simulink model "FullState_HOSMO_UKF_STC_Half_Car_02_noised"  (R2022a)
settings: Solver=ode4  StartTime=0.0  StopTime=5  FixedStep=1e-4  RelTol=1e-3
undefined symbols (not defined in the file): DiscIntNeverNeededParam
libraries: simulink x5, sharedTrackingLibrary x1
settings Model: Creator=user  LastModifiedBy=user

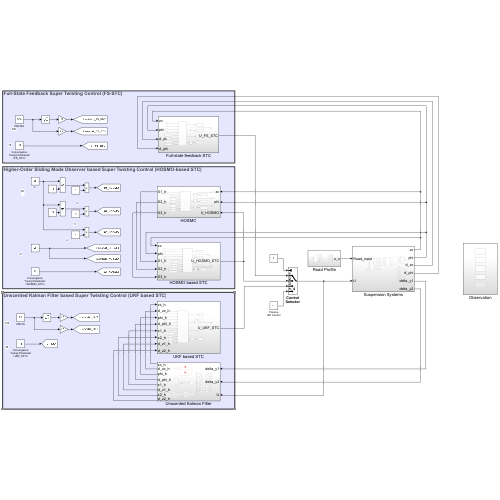
[thumbnail: Simulink's stored preview of the top-level diagram]
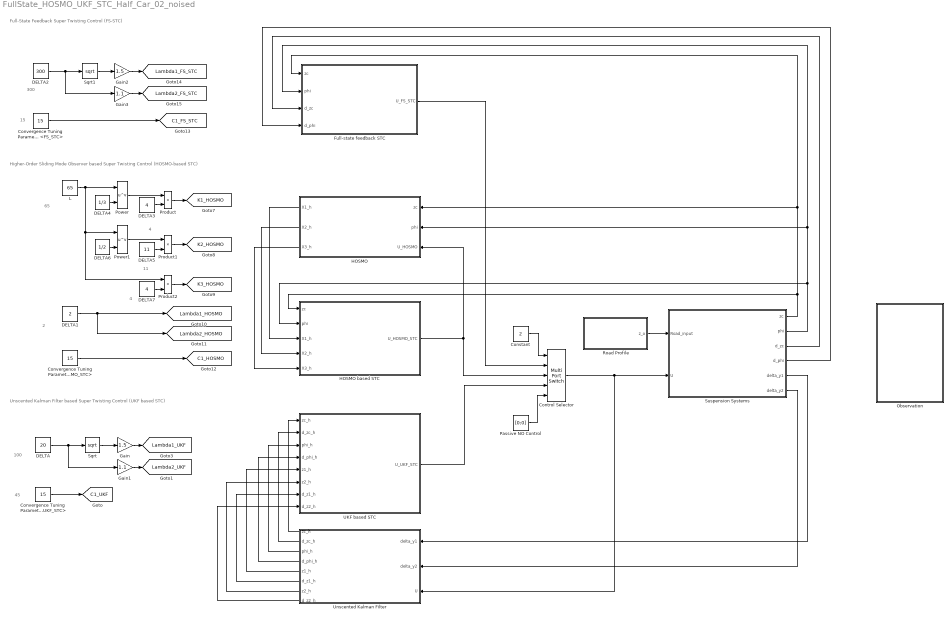
== system FullState_HOSMO_UKF_STC_Half_Car_02_noised ==
  note: 4
  note: 11
  note: 4
  note: 45
  note: 100
  note: 15
  note: 300
  note: 2
  note: 65
  note: Unscented Kalman Filter based Super Twisting Control (UKF based STC)
  note: Higher-Order Sliding Mode Observer based Super Twisting Control (HOSMO-based STC)
  note: Full-State Feedback Super Twisting Control (FS-STC)
  Constant : Constant  Value=2
  Control Selector : MultiPortSwitch  Inputs=4  SaturateOnIntegerOverflow=off  InputSameDT=off
  Convergence Tuning Parameter <FS_STC> : Constant  Value=15
  Convergence Tuning Parameter <HOSMO_STC> : Constant  Value=15
  Convergence Tuning Parameter <UKF_STC> : Constant  Value=15
  DELTA : Constant  Value=20
  DELTA1 : Constant  Value=2
  DELTA2 : Constant  Value=300
  DELTA3 : Constant  Value=4
  DELTA4 : Constant  Value=1/3
  DELTA5 : Constant  Value=11
  DELTA6 : Constant  Value=1/2
  DELTA7 : Constant  Value=4
  Full-state feedback STC : Subsystem
  Gain : Gain  Gain=1.5
  Gain1 : Gain  Gain=1.1
  Gain2 : Gain  Gain=1.5
  Gain3 : Gain  Gain=1.1
  HOSMO : Subsystem
  HOSMO based STC : Subsystem
  L : Constant  Value=65
  Observation : Subsystem
  Passive NO Control : Constant  Value=[0;0]
  Power : Math  Operator=pow
  Power1 : Math  Operator=pow
  Product : Product
  Product1 : Product
  Product2 : Product
  Road Profile : Subsystem
  Sqrt : Sqrt
  Sqrt1 : Sqrt
  Suspension Systems : Subsystem
  UKF based STC : Subsystem
  Unscented Kalman Filter : Subsystem
  tag scope: C1_FS_STC=global, C1_HOSMO=global, C1_UKF=global, K1_HOSMO=global, K2_HOSMO=global, K3_HOSMO=global, Lambda1_FS_STC=global, Lambda1_HOSMO=global, Lambda1_UKF=global, Lambda2_FS_STC=global, Lambda2_HOSMO=global, Lambda2_UKF=global
  wires:
  Road Profile/1(z_o) -> Suspension Systems/1(Road_input)
  Suspension Systems/5(delta_y1) -> Unscented Kalman Filter/1(delta_y1)
  Suspension Systems/6(delta_y2) -> Unscented Kalman Filter/2(delta_y2)
  Control Selector/1 -> Unscented Kalman Filter/3(U), Suspension Systems/2(U)
  Unscented Kalman Filter/1(zc_h) -> UKF based STC/1(zc_h)
  Unscented Kalman Filter/2(d_zc_h) -> UKF based STC/2(d_zc_h)
  Unscented Kalman Filter/3(phi_h) -> UKF based STC/3(phi_h)
  Unscented Kalman Filter/4(d_phi_h) -> UKF based STC/4(d_phi_h)
  Unscented Kalman Filter/6(d_z1_h) -> UKF based STC/7(d_z1_h)
  Unscented Kalman Filter/8(d_z2_h) -> UKF based STC/8(d_z2_h)
  Unscented Kalman Filter/7(z2_h) -> UKF based STC/6(z2_h)
  Unscented Kalman Filter/5(z1_h) -> UKF based STC/5(z1_h)
  Constant/1 -> Control Selector/1
  Passive NO Control/1 -> Control Selector/5
  UKF based STC/1(U_UKF_STC) -> Control Selector/4
  HOSMO based STC/1(U_HOSMO_STC) -> Control Selector/3, HOSMO/3(U_HOSMO)
  HOSMO/1(X1_h) -> HOSMO based STC/3(X1_h)
  HOSMO/2(X2_h) -> HOSMO based STC/4(X2_h)
  HOSMO/3(X3_h) -> HOSMO based STC/5(X3_h)
  Suspension Systems/1(zc) -> Full-state feedback STC/1(zc), HOSMO/1(zc), HOSMO based STC/1(zc)
  Suspension Systems/2(phi) -> Full-state feedback STC/2(phi), HOSMO/2(phi), HOSMO based STC/2(phi)
  DELTA/1 -> Sqrt/1, Gain1/1
  Convergence Tuning Parameter <UKF_STC>/1 -> [C1_UKF]
  Gain/1 -> [Lambda1_UKF]
  Gain1/1 -> [Lambda2_UKF]
  Sqrt/1 -> Gain/1
  Convergence Tuning Parameter <HOSMO_STC>/1 -> [C1_HOSMO]
  DELTA1/1 -> [Lambda2_HOSMO], [Lambda1_HOSMO]
  L/1 -> Product2/1, Power1/1, Power/1
  Product/1 -> [K1_HOSMO]
  DELTA4/1 -> Power/2
  Power/1 -> Product/1
  DELTA3/1 -> Product/2
  DELTA5/1 -> Product1/2
  Power1/1 -> Product1/1
  DELTA6/1 -> Power1/2
  Product1/1 -> [K2_HOSMO]
  DELTA7/1 -> Product2/2
  Product2/1 -> [K3_HOSMO]
  Convergence Tuning Parameter <FS_STC>/1 -> [C1_FS_STC]
  Sqrt1/1 -> Gain2/1
  DELTA2/1 -> Sqrt1/1, Gain3/1
  Gain2/1 -> [Lambda1_FS_STC]
  Gain3/1 -> [Lambda2_FS_STC]
  Full-state feedback STC/1(U_FS_STC) -> Control Selector/2
  Suspension Systems/3(d_zc) -> Full-state feedback STC/3(d_zc)
  Suspension Systems/4(d_phi) -> Full-state feedback STC/4(d_phi)

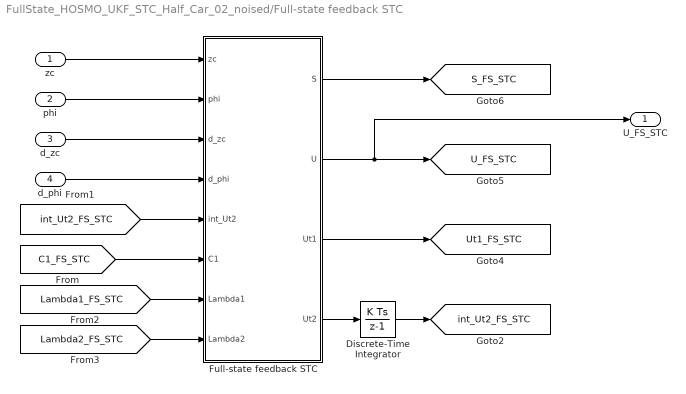
== system FullState_HOSMO_UKF_STC_Half_Car_02_noised/Full-state feedback STC ==
  zc : Inport
  phi : Inport  Port=2
  d_zc : Inport  Port=3
  d_phi : Inport  Port=4
  Discrete-Time Integrator : DiscreteIntegrator  InitialCondition=[0;0]  SampleTime=-1  ICPrevOutput=DiscIntNeverNeededParam  ICPrevScaledInput=DiscIntNeverNeededParam
  Full-state feedback STC : MATLAB Function  TreatAsAtomicUnit=on
  U_FS_STC : Outport
  tag scope: S_FS_STC=global, U_FS_STC=global, Ut1_FS_STC=global, int_Ut2_FS_STC=global
  wires:
  d_phi/1 -> Full-state feedback STC/4(d_phi)
  d_zc/1 -> Full-state feedback STC/3(d_zc)
  Full-state feedback STC/3(Ut1) -> [Ut1_FS_STC]
  [Lambda2_FS_STC] -> Full-state feedback STC/8(Lambda2)
  zc/1 -> Full-state feedback STC/1(zc)
  Discrete-Time Integrator/1 -> [int_Ut2_FS_STC]
  Full-state feedback STC/4(Ut2) -> Discrete-Time Integrator/1
  Full-state feedback STC/2(U) -> U_FS_STC/1, [U_FS_STC]
  phi/1 -> Full-state feedback STC/2(phi)
  Full-state feedback STC/1(S) -> [S_FS_STC]
  [Lambda1_FS_STC] -> Full-state feedback STC/7(Lambda1)
  [int_Ut2_FS_STC] -> Full-state feedback STC/5(int_Ut2)
  [C1_FS_STC] -> Full-state feedback STC/6(C1)

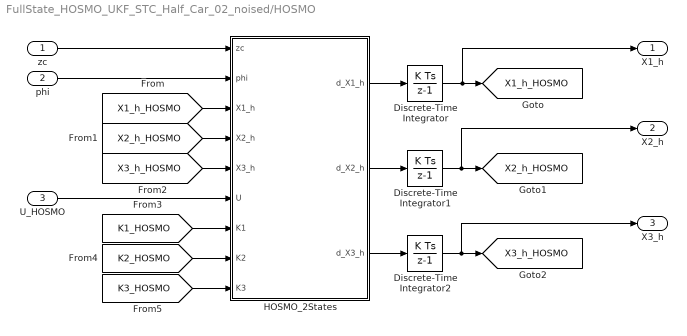
== system FullState_HOSMO_UKF_STC_Half_Car_02_noised/HOSMO ==
  zc : Inport
  phi : Inport  Port=2
  U_HOSMO : Inport  Port=3
  Discrete-Time Integrator : DiscreteIntegrator  InitialCondition=[0;0]  SampleTime=-1  ICPrevOutput=DiscIntNeverNeededParam  ICPrevScaledInput=DiscIntNeverNeededParam
  Discrete-Time Integrator1 : DiscreteIntegrator  InitialCondition=[0;0]  SampleTime=-1  ICPrevOutput=DiscIntNeverNeededParam  ICPrevScaledInput=DiscIntNeverNeededParam
  Discrete-Time Integrator2 : DiscreteIntegrator  InitialCondition=[0;0]  SampleTime=-1  ICPrevOutput=DiscIntNeverNeededParam  ICPrevScaledInput=DiscIntNeverNeededParam
  HOSMO_2States : MATLAB Function  TreatAsAtomicUnit=on
  X1_h : Outport
  X2_h : Outport  Port=2
  X3_h : Outport  Port=3
  tag scope: X1_h_HOSMO=global, X2_h_HOSMO=global, X3_h_HOSMO=global
  wires:
  HOSMO_2States/2(d_X2_h) -> Discrete-Time Integrator1/1
  [K1_HOSMO] -> HOSMO_2States/7(K1)
  Discrete-Time Integrator1/1 -> X2_h/1, [X2_h_HOSMO]
  [K2_HOSMO] -> HOSMO_2States/8(K2)
  [K3_HOSMO] -> HOSMO_2States/9(K3)
  [X1_h_HOSMO] -> HOSMO_2States/3(X1_h)
  [X3_h_HOSMO] -> HOSMO_2States/5(X3_h)
  Discrete-Time Integrator/1 -> X1_h/1, [X1_h_HOSMO]
  HOSMO_2States/1(d_X1_h) -> Discrete-Time Integrator/1
  HOSMO_2States/3(d_X3_h) -> Discrete-Time Integrator2/1
  zc/1 -> HOSMO_2States/1(zc)
  [X2_h_HOSMO] -> HOSMO_2States/4(X2_h)
  Discrete-Time Integrator2/1 -> X3_h/1, [X3_h_HOSMO]
  phi/1 -> HOSMO_2States/2(phi)
  U_HOSMO/1 -> HOSMO_2States/6(U)

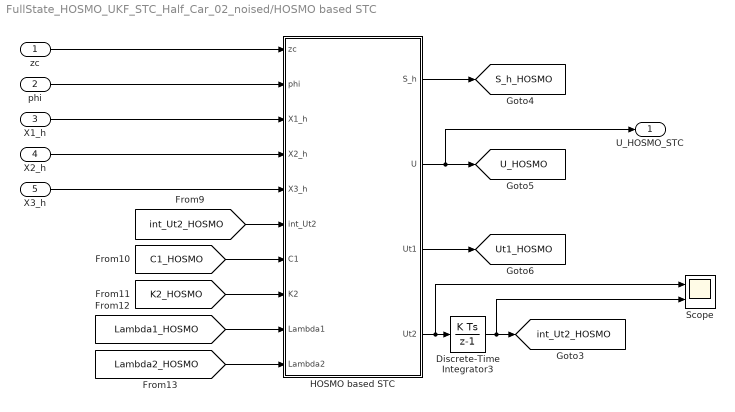
== system FullState_HOSMO_UKF_STC_Half_Car_02_noised/HOSMO based STC ==
  zc : Inport
  phi : Inport  Port=2
  X1_h : Inport  Port=3
  X2_h : Inport  Port=4
  X3_h : Inport  Port=5
  Discrete-Time Integrator3 : DiscreteIntegrator  InitialCondition=[0;0]  SampleTime=-1  ICPrevOutput=DiscIntNeverNeededParam  ICPrevScaledInput=DiscIntNeverNeededParam
  HOSMO based STC : MATLAB Function  TreatAsAtomicUnit=on
  Scope : Scope  NumInputPorts=2
  U_HOSMO_STC : Outport
  tag scope: S_h_HOSMO=global, U_HOSMO=global, Ut1_HOSMO=global, int_Ut2_HOSMO=global
  wires:
  Discrete-Time Integrator3/1 -> Scope/2, [int_Ut2_HOSMO]
  [Lambda1_HOSMO] -> HOSMO based STC/9(Lambda1)
  HOSMO based STC/1(S_h) -> [S_h_HOSMO]
  HOSMO based STC/2(U) -> U_HOSMO_STC/1, [U_HOSMO]
  HOSMO based STC/3(Ut1) -> [Ut1_HOSMO]
  X3_h/1 -> HOSMO based STC/5(X3_h)
  [Lambda2_HOSMO] -> HOSMO based STC/10(Lambda2)
  X1_h/1 -> HOSMO based STC/3(X1_h)
  phi/1 -> HOSMO based STC/2(phi)
  X2_h/1 -> HOSMO based STC/4(X2_h)
  [int_Ut2_HOSMO] -> HOSMO based STC/6(int_Ut2)
  [K2_HOSMO] -> HOSMO based STC/8(K2)
  [C1_HOSMO] -> HOSMO based STC/7(C1)
  HOSMO based STC/4(Ut2) -> Scope/1, Discrete-Time Integrator3/1
  zc/1 -> HOSMO based STC/1(zc)

== system FullState_HOSMO_UKF_STC_Half_Car_02_noised/Observation ==
  FullState_STC : Subsystem
  HOSMO_STC : Subsystem
  OVERALL : Subsystem
  To Workspace : Subsystem  Commented=on
  UKF_STC : Subsystem

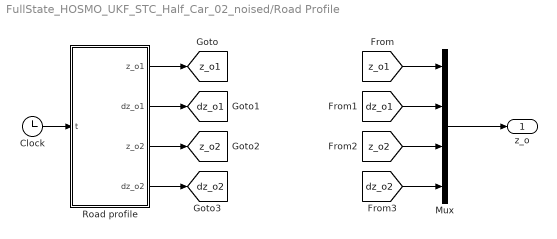
== system FullState_HOSMO_UKF_STC_Half_Car_02_noised/Road Profile ==
  Clock : Clock
  Mux : Mux
  Road profile : MATLAB Function  TreatAsAtomicUnit=on
  z_o : Outport
  tag scope: dz_o1=global, dz_o2=global, z_o1=global, z_o2=global
  wires:
  Road profile/3(z_o2) -> [z_o2]
  Mux/1 -> z_o/1
  Road profile/1(z_o1) -> [z_o1]
  Clock/1 -> Road profile/1(t)
  Road profile/4(dz_o2) -> [dz_o2]
  Road profile/2(dz_o1) -> [dz_o1]
  [z_o1] -> Mux/1
  [dz_o1] -> Mux/2
  [dz_o2] -> Mux/4
  [z_o2] -> Mux/3

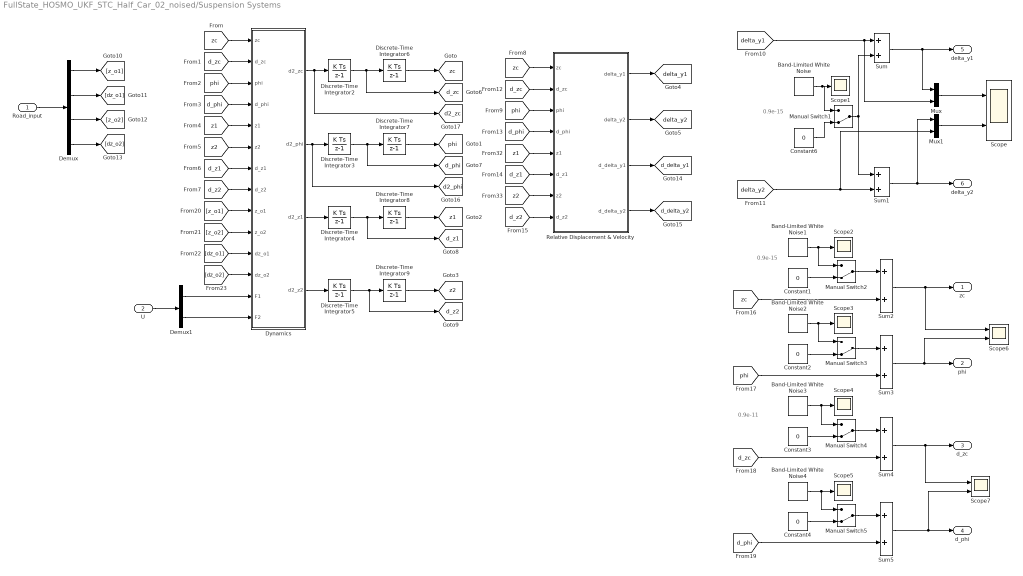
== system FullState_HOSMO_UKF_STC_Half_Car_02_noised/Suspension Systems ==
  note: 0.9e-11
  note: 0.9e-15
  note: 0.9e-15
  Road_input : Inport
  U : Inport  Port=2
  Band-Limited White Noise : simulink/Sources/Band-Limited White Noise  Cov=0.9e-15  Ts=1e-4  seed=[23341]
  Band-Limited White Noise1 : simulink/Sources/Band-Limited White Noise  Cov=0.9e-15  Ts=1e-4  seed=[23341]
  Band-Limited White Noise2 : simulink/Sources/Band-Limited White Noise  Cov=0.9e-15  Ts=1e-4  seed=[23341]
  Band-Limited White Noise3 : simulink/Sources/Band-Limited White Noise  Cov=0.9e-11  Ts=1e-4  seed=[23341]
  Band-Limited White Noise4 : simulink/Sources/Band-Limited White Noise  Cov=0.9e-11  Ts=1e-4  seed=[23341]
  Constant{1..4,6} (5 alike) : Constant  Value=0
  Demux : Demux
  Demux1 : Demux  Outputs=2
  Discrete-Time Integrator{2..9} (8 alike) : DiscreteIntegrator  SampleTime=-1  ICPrevOutput=DiscIntNeverNeededParam  ICPrevScaledInput=DiscIntNeverNeededParam
  Dynamics : MATLAB Function  TreatAsAtomicUnit=on
  Manual Switch{1..5} (5 alike) : ManualSwitch  CurrentSetting=0
  Mux : Mux  Inputs=2
  Mux1 : Mux  Inputs=2
  Relative Displacement & Velocity : MATLAB Function  TreatAsAtomicUnit=on
  Scope : Scope  NumInputPorts=2
  Scope{1..5} (5 alike) : Scope
  Scope6 : Scope  NumInputPorts=2
  Scope7 : Scope  NumInputPorts=2
  Sum{,1..5} (6 alike) : Sum
  zc : Outport
  phi : Outport  Port=2
  d_zc : Outport  Port=3
  d_phi : Outport  Port=4
  delta_y1 : Outport  Port=5
  delta_y2 : Outport  Port=6
  tag scope: d2_phi=global, d2_zc=global, d_delta_y1=global, d_delta_y2=global, d_phi=global, d_z1=global, d_z2=global, d_zc=global, delta_y1=global, delta_y2=global, phi=global, z1=global, z2=global, zc=global
  wires:
  Dynamics/4(d2_z2) -> Discrete-Time Integrator5/1
  Discrete-Time Integrator2/1 -> [d_zc], Discrete-Time Integrator6/1
  Relative Displacement & Velocity/1(delta_y1) -> [delta_y1]
  Discrete-Time Integrator4/1 -> [d_z1], Discrete-Time Integrator8/1
  [z1] -> Dynamics/5(z1)
  [dz_o2] -> Dynamics/12(dz_o2)
  Discrete-Time Integrator3/1 -> [d_phi], Discrete-Time Integrator7/1
  [zc] -> Relative Displacement & Velocity/1(zc)
  Dynamics/2(d2_phi) -> [d2_phi], Discrete-Time Integrator3/1
  [d_phi] -> Dynamics/4(d_phi)
  Discrete-Time Integrator5/1 -> [d_z2], Discrete-Time Integrator9/1
  Discrete-Time Integrator7/1 -> [phi]
  [z_o2] -> Dynamics/10(z_o2)
  [z1] -> Relative Displacement & Velocity/5(z1)
  Discrete-Time Integrator6/1 -> [zc]
  Dynamics/3(d2_z1) -> Discrete-Time Integrator4/1
  Discrete-Time Integrator8/1 -> [z1]
  [d_zc] -> Dynamics/2(d_zc)
  [phi] -> Dynamics/3(phi)
  Road_input/1 -> Demux/1
  [z2] -> Dynamics/6(z2)
  [zc] -> Dynamics/1(zc)
  [z_o1] -> Dynamics/9(z_o1)
  Dynamics/1(d2_zc) -> [d2_zc], Discrete-Time Integrator2/1
  [d_z1] -> Dynamics/7(d_z1)
  [dz_o1] -> Dynamics/11(dz_o1)
  Relative Displacement & Velocity/2(delta_y2) -> [delta_y2]
  [d_z2] -> Dynamics/8(d_z2)
  Discrete-Time Integrator9/1 -> [z2]
  [phi] -> Relative Displacement & Velocity/3(phi)
  [z2] -> Relative Displacement & Velocity/7(z2)
  Demux/1 -> [z_o1]
  Demux/2 -> [dz_o1]
  Demux/3 -> [z_o2]
  Demux/4 -> [dz_o2]
  [d_zc] -> Relative Displacement & Velocity/2(d_zc)
  [d_phi] -> Relative Displacement & Velocity/4(d_phi)
  [d_z1] -> Relative Displacement & Velocity/6(d_z1)
  [d_z2] -> Relative Displacement & Velocity/8(d_z2)
  Relative Displacement & Velocity/3(d_delta_y1) -> [d_delta_y1]
  Relative Displacement & Velocity/4(d_delta_y2) -> [d_delta_y2]
  Demux1/1 -> Dynamics/13(F1)
  Demux1/2 -> Dynamics/14(F2)
  U/1 -> Demux1/1
  Manual Switch1/1 -> Sum1/1, Sum/2
  Constant6/1 -> Manual Switch1/2
  Sum1/1 -> Mux1/1, delta_y2/1
  Sum/1 -> Mux/1, delta_y1/1
  [delta_y1] -> Sum/1, Mux/2
  Band-Limited White Noise/1 -> Manual Switch1/1, Scope1/1
  [delta_y2] -> Mux1/2, Sum1/2
  Mux/1 -> Scope/1
  Mux1/1 -> Scope/2
  [zc] -> Sum2/2
  Band-Limited White Noise1/1 -> Manual Switch2/1, Scope2/1
  Constant1/1 -> Manual Switch2/2
  Manual Switch2/1 -> Sum2/1
  Sum2/1 -> Scope6/1, zc/1
  Sum3/1 -> Scope6/2, phi/1
  Manual Switch3/1 -> Sum3/1
  Constant2/1 -> Manual Switch3/2
  Band-Limited White Noise2/1 -> Scope3/1, Manual Switch3/1
  [phi] -> Sum3/2
  Band-Limited White Noise3/1 -> Scope4/1, Manual Switch4/1
  Constant3/1 -> Manual Switch4/2
  Manual Switch4/1 -> Sum4/1
  [d_zc] -> Sum4/2
  Sum4/1 -> Scope7/1, d_zc/1
  Manual Switch5/1 -> Sum5/1
  Constant4/1 -> Manual Switch5/2
  Band-Limited White Noise4/1 -> Manual Switch5/1, Scope5/1
  [d_phi] -> Sum5/2
  Sum5/1 -> Scope7/2, d_phi/1

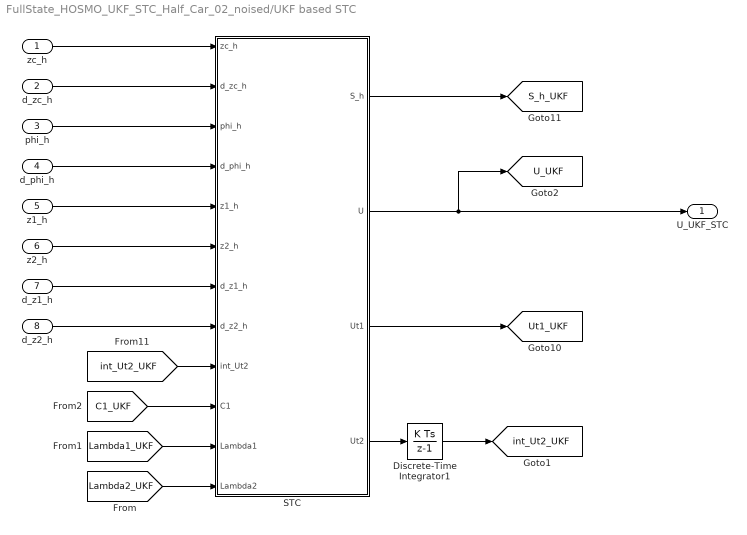
== system FullState_HOSMO_UKF_STC_Half_Car_02_noised/UKF based STC ==
  zc_h : Inport
  d_zc_h : Inport  Port=2
  phi_h : Inport  Port=3
  d_phi_h : Inport  Port=4
  z1_h : Inport  Port=5
  z2_h : Inport  Port=6
  d_z1_h : Inport  Port=7
  d_z2_h : Inport  Port=8
  Discrete-Time Integrator1 : DiscreteIntegrator  InitialCondition=[0;0]  SampleTime=-1  ICPrevOutput=DiscIntNeverNeededParam  ICPrevScaledInput=DiscIntNeverNeededParam
  STC : MATLAB Function  TreatAsAtomicUnit=on
  U_UKF_STC : Outport
  tag scope: S_h_UKF=global, U_UKF=global, Ut1_UKF=global, int_Ut2_UKF=global
  wires:
  phi_h/1 -> STC/3(phi_h)
  STC/2(U) -> [U_UKF], U_UKF_STC/1
  d_zc_h/1 -> STC/2(d_zc_h)
  zc_h/1 -> STC/1(zc_h)
  z2_h/1 -> STC/6(z2_h)
  [Lambda2_UKF] -> STC/12(Lambda2)
  Discrete-Time Integrator1/1 -> [int_Ut2_UKF]
  STC/1(S_h) -> [S_h_UKF]
  z1_h/1 -> STC/5(z1_h)
  STC/3(Ut1) -> [Ut1_UKF]
  [Lambda1_UKF] -> STC/11(Lambda1)
  [C1_UKF] -> STC/10(C1)
  STC/4(Ut2) -> Discrete-Time Integrator1/1
  d_phi_h/1 -> STC/4(d_phi_h)
  [int_Ut2_UKF] -> STC/9(int_Ut2)
  d_z1_h/1 -> STC/7(d_z1_h)
  d_z2_h/1 -> STC/8(d_z2_h)

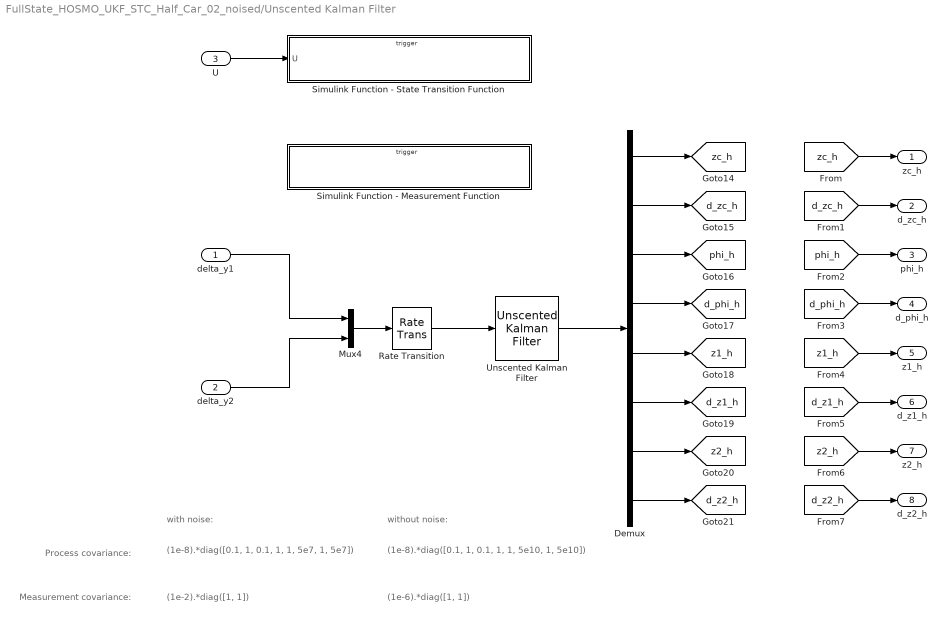
== system FullState_HOSMO_UKF_STC_Half_Car_02_noised/Unscented Kalman Filter ==
  note: Measurement covariance:
  note: (1e-6).*diag([1, 1])
  note: (1e-8).*diag([0.1, 1, 0.1, 1, 1, 5e7, 1, 5e7])
  note: (1e-2).*diag([1, 1])
  note: Process covariance:
  note: with noise:
  note: without noise:
  note: (1e-8).*diag([0.1, 1, 0.1, 1, 1, 5e10, 1, 5e10])
  delta_y1 : Inport
  delta_y2 : Inport  Port=2
  U : Inport  Port=3
  Demux : Demux  Outputs=8
  Mux4 : Mux  Inputs=2
  Rate Transition : RateTransition  InitialCondition=[0;0]  OutPortSampleTime=1e-4
  Simulink Function - Measurement Function : Subsystem  TreatAsAtomicUnit=on
  Simulink Function - State Transition Function : Subsystem  TreatAsAtomicUnit=on
  Unscented Kalman Filter : sharedTrackingLibrary/Unscented Kalman Filter  StateTransitionFcn=SuspensionStateFcn  HasAdditiveProcessNoise=Additive  ProcessNoise=(1e-8).*diag([0.1, 1, 0.1, 1, 1, 5e10, 1, 5e10])  HasTimeVaryingProcessNoise=off  HasStateTransitionFcnExtraArgument=0  InitialState=zeros(8,1)  InitialStateCovariance=diag([0, 0, 0, 0, 0, 0, 0, 0])  Alpha=1  Beta=2  Kappa=0  MeasurementFcn1=SuspensionMeasurementFcn  HasMeasurementEnablePort1=off  HasAdditiveMeasurementNoise1=Additive  MeasurementNoise1=(1e-6).*diag([1, 1])  HasTimeVaryingMeasurementNoise1=off  HasMeasurementFcnExtraArgument1=0  HasMeasurementWrapping1=off  MeasurementFcn2=myMeasurementFcn  HasMeasurementEnablePort2=off  HasAdditiveMeasurementNoise2=Additive  MeasurementNoise2=1  HasTimeVaryingMeasurementNoise2=off  HasMeasurementFcnExtraArgument2=0  HasMeasurementWrapping2=off  MeasurementFcn3=myMeasurementFcn  HasMeasurementEnablePort3=off  HasAdditiveMeasurementNoise3=Additive  MeasurementNoise3=1  HasTimeVaryingMeasurementNoise3=off  HasMeasurementFcnExtraArgument3=0  HasMeasurementWrapping3=off  MeasurementFcn4=myMeasurementFcn  HasMeasurementEnablePort4=off  HasAdditiveMeasurementNoise4=Additive  MeasurementNoise4=1  HasTimeVaryingMeasurementNoise4=off  HasMeasurementFcnExtraArgument4=0  HasMeasurementWrapping4=off  MeasurementFcn5=myMeasurementFcn  HasMeasurementEnablePort5=off  HasAdditiveMeasurementNoise5=Additive  MeasurementNoise5=1  HasTimeVaryingMeasurementNoise5=off  HasMeasurementFcnExtraArgument5=0  HasMeasurementWrapping5=off  EnableMultirate=off  StateTransitionFcnSampleTime=-1  MeasurementFcn1SampleTime=-1  MeasurementFcn2SampleTime=-1  MeasurementFcn3SampleTime=-1  MeasurementFcn4SampleTime=-1  MeasurementFcn5SampleTime=-1  UseCurrentEstimator=on  OutputStateCovariance=off  DataType=double  SampleTime=1e-4  NumberOfMeasurements=1
      settings: SourceProductBaseCode=TF,AE,PW,CT,DR,ID,LP,NV,AR,RO,RR,UV,VE
  zc_h : Outport
  d_zc_h : Outport  Port=2
  phi_h : Outport  Port=3
  d_phi_h : Outport  Port=4
  z1_h : Outport  Port=5
  d_z1_h : Outport  Port=6
  z2_h : Outport  Port=7
  d_z2_h : Outport  Port=8
  tag scope: d_phi_h=global, d_z1_h=global, d_z2_h=global, d_zc_h=global, phi_h=global, z1_h=global, z2_h=global, zc_h=global
  wires:
  Mux4/1 -> Rate Transition/1
  Demux/4 -> [d_phi_h]
  U/1 -> Simulink Function - State Transition Function/1(U)
  Demux/8 -> [d_z2_h]
  Unscented Kalman Filter/1 -> Demux/1
  Rate Transition/1 -> Unscented Kalman Filter/1
  Demux/6 -> [d_z1_h]
  Demux/5 -> [z1_h]
  Demux/2 -> [d_zc_h]
  Demux/7 -> [z2_h]
  Demux/1 -> [zc_h]
  Demux/3 -> [phi_h]
  [d_z2_h] -> d_z2_h/1
  [d_z1_h] -> d_z1_h/1
  [d_phi_h] -> d_phi_h/1
  [phi_h] -> phi_h/1
  [d_zc_h] -> d_zc_h/1
  [zc_h] -> zc_h/1
  [z1_h] -> z1_h/1
  [z2_h] -> z2_h/1
  delta_y1/1 -> Mux4/1
  delta_y2/1 -> Mux4/2

== system FullState_HOSMO_UKF_STC_Half_Car_02_noised/Observation/FullState_STC ==
  FS_STC : Scope  NumInputPorts=4
  wires:
  [Ut1_FS_STC] -> FS_STC/3  "Super twisting control 1"
  [U_FS_STC] -> FS_STC/2  "Total Control"
  [int_Ut2_FS_STC] -> FS_STC/4  "Super twisting control 2"
  [S_FS_STC] -> FS_STC/1  "Sliding Surface"

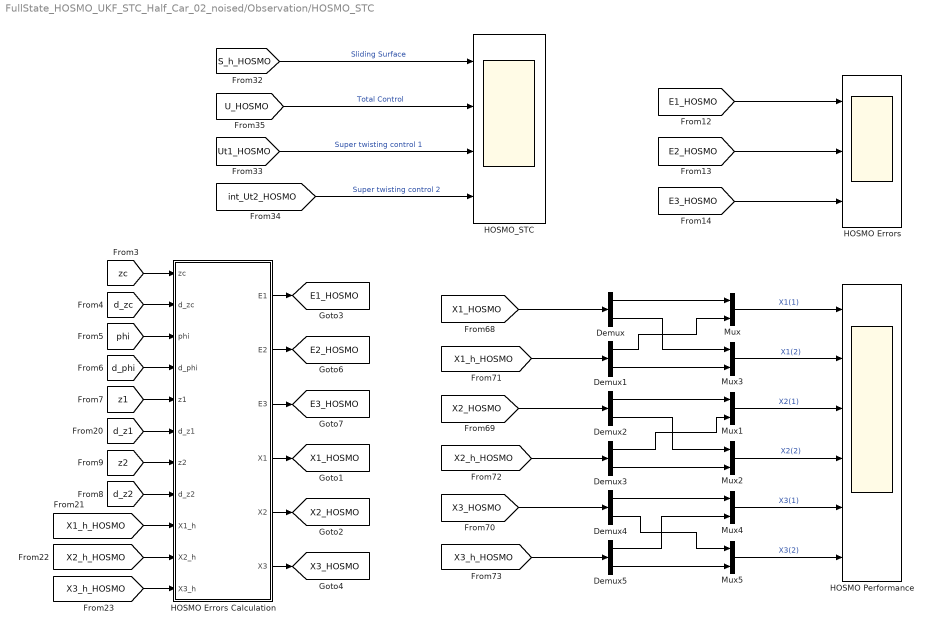
== system FullState_HOSMO_UKF_STC_Half_Car_02_noised/Observation/HOSMO_STC ==
  Demux{,1..5} (6 alike) : Demux  Outputs=2
  HOSMO Errors : Scope  NumInputPorts=3
  HOSMO Errors Calculation : MATLAB Function  TreatAsAtomicUnit=on
  HOSMO Performance : Scope  NumInputPorts=6
  HOSMO_STC : Scope  NumInputPorts=4
  Mux{,1..5} (6 alike) : Mux  Inputs=2
  tag scope: E1_HOSMO=global, E2_HOSMO=global, E3_HOSMO=global, X1_HOSMO=global, X2_HOSMO=global, X3_HOSMO=global
  wires:
  Demux1/2 -> Mux3/2
  HOSMO Errors Calculation/6(X3) -> [X3_HOSMO]
  Demux/1 -> Mux/1
  Demux5/1 -> Mux4/2
  [d_phi] -> HOSMO Errors Calculation/4(d_phi)
  [X2_HOSMO] -> Demux2/1
  HOSMO Errors Calculation/2(E2) -> [E2_HOSMO]
  Mux5/1 -> HOSMO Performance/6  "X3(2)"
  [X3_h_HOSMO] -> HOSMO Errors Calculation/11(X3_h)
  Demux/2 -> Mux3/1
  [d_z1] -> HOSMO Errors Calculation/6(d_z1)
  [d_z2] -> HOSMO Errors Calculation/8(d_z2)
  HOSMO Errors Calculation/4(X1) -> [X1_HOSMO]
  Demux2/1 -> Mux1/1
  [d_zc] -> HOSMO Errors Calculation/2(d_zc)
  HOSMO Errors Calculation/3(E3) -> [E3_HOSMO]
  [X2_h_HOSMO] -> Demux3/1
  [X1_HOSMO] -> Demux/1
  Demux2/2 -> Mux2/1
  HOSMO Errors Calculation/5(X2) -> [X2_HOSMO]
  [X3_h_HOSMO] -> Demux5/1
  Mux/1 -> HOSMO Performance/1  "X1(1)"
  Demux4/2 -> Mux5/1
  HOSMO Errors Calculation/1(E1) -> [E1_HOSMO]
  Demux4/1 -> Mux4/1
  [int_Ut2_HOSMO] -> HOSMO_STC/4  "Super twisting control 2"
  Demux5/2 -> Mux5/2
  [X1_h_HOSMO] -> Demux1/1
  [z2] -> HOSMO Errors Calculation/7(z2)
  Mux3/1 -> HOSMO Performance/2  "X1(2)"
  Mux1/1 -> HOSMO Performance/3  "X2(1)"
  Mux4/1 -> HOSMO Performance/5  "X3(1)"
  Demux3/2 -> Mux2/2
  Mux2/1 -> HOSMO Performance/4  "X2(2)"
  [U_HOSMO] -> HOSMO_STC/2  "Total Control"
  [X1_h_HOSMO] -> HOSMO Errors Calculation/9(X1_h)
  [E3_HOSMO] -> HOSMO Errors/3
  [S_h_HOSMO] -> HOSMO_STC/1  "Sliding Surface"
  [X3_HOSMO] -> Demux4/1
  [X2_h_HOSMO] -> HOSMO Errors Calculation/10(X2_h)
  Demux1/1 -> Mux/2
  [phi] -> HOSMO Errors Calculation/3(phi)
  [zc] -> HOSMO Errors Calculation/1(zc)
  [Ut1_HOSMO] -> HOSMO_STC/3  "Super twisting control 1"
  [z1] -> HOSMO Errors Calculation/5(z1)
  [E2_HOSMO] -> HOSMO Errors/2
  Demux3/1 -> Mux1/2
  [E1_HOSMO] -> HOSMO Errors/1

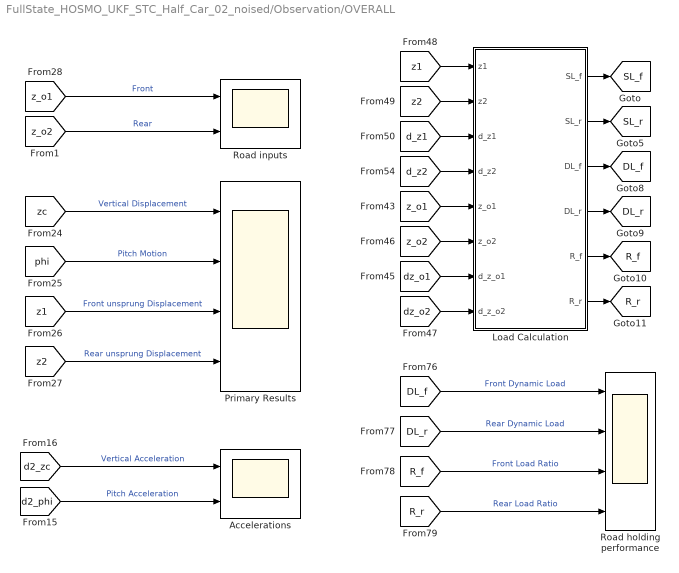
== system FullState_HOSMO_UKF_STC_Half_Car_02_noised/Observation/OVERALL ==
  Accelerations : Scope  NumInputPorts=2
  Load Calculation : MATLAB Function  TreatAsAtomicUnit=on
  Primary Results : Scope  NumInputPorts=4
  Road holding performance : Scope  NumInputPorts=4
  Road inputs : Scope  NumInputPorts=2
  tag scope: DL_f=global, DL_r=global, R_f=global, R_r=global, SL_f=global, SL_r=global
  wires:
  Load Calculation/2(SL_r) -> [SL_r]
  [DL_f] -> Road holding performance/1  "Front Dynamic Load"
  [z_o2] -> Load Calculation/6(z_o2)
  Load Calculation/6(R_r) -> [R_r]
  [z_o1] -> Load Calculation/5(z_o1)
  [d_z1] -> Load Calculation/3(d_z1)
  Load Calculation/5(R_f) -> [R_f]
  [d2_phi] -> Accelerations/2  "Pitch Acceleration"
  Load Calculation/3(DL_f) -> [DL_f]
  [zc] -> Primary Results/1  "Vertical Displacement"
  [d_z2] -> Load Calculation/4(d_z2)
  [z1] -> Load Calculation/1(z1)
  [z2] -> Load Calculation/2(z2)
  [d2_zc] -> Accelerations/1  "Vertical Acceleration"
  Load Calculation/1(SL_f) -> [SL_f]
  [z2] -> Primary Results/4  "Rear unsprung Displacement"
  [z1] -> Primary Results/3  "Front unsprung Displacement"
  [dz_o1] -> Load Calculation/7(d_z_o1)
  [R_f] -> Road holding performance/3  "Front Load Ratio"
  [phi] -> Primary Results/2  "Pitch Motion"
  [dz_o2] -> Load Calculation/8(d_z_o2)
  Load Calculation/4(DL_r) -> [DL_r]
  [z_o1] -> Road inputs/1  "Front"
  [R_r] -> Road holding performance/4  "Rear Load Ratio"
  [z_o2] -> Road inputs/2  "Rear"
  [DL_r] -> Road holding performance/2  "Rear Dynamic Load"

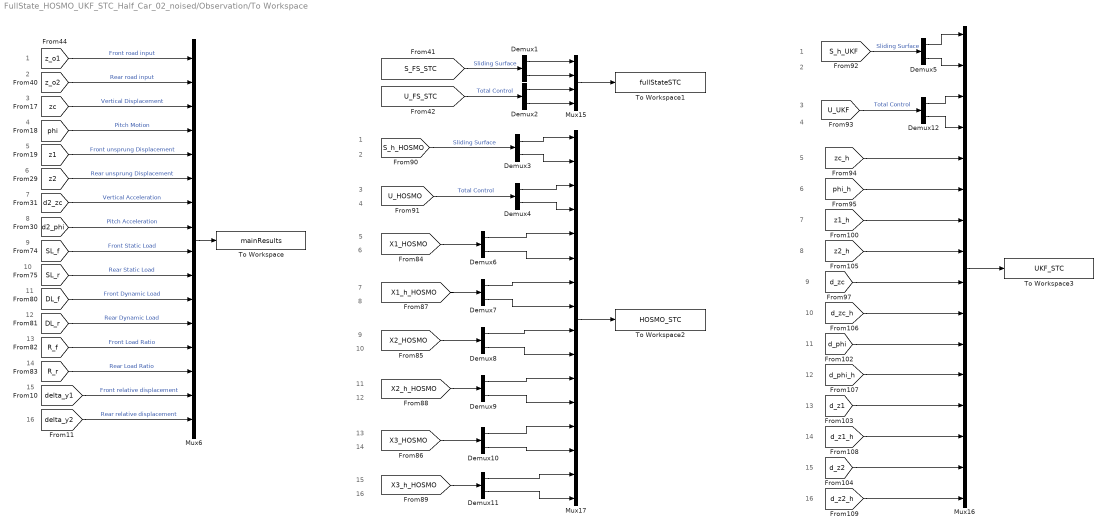
== system FullState_HOSMO_UKF_STC_Half_Car_02_noised/Observation/To Workspace ==
  note: 16
  note: 15
  note: 14
  note: 13
  note: 12
  note: 11
  note: 10
  note: 9
  note: 8
  note: 7
  note: 6
  note: 5
  note: 4
  note: 3
  note: 2
  note: 1
  note: 9
  note: 13
  note: 8
  note: 6
  note: 2
  note: 12
  note: 3
  note: 16
  note: 11
  note: 10
  note: 14
  note: 7
  note: 5
  note: 15
  note: 4
  note: 1
  note: 9
  note: 13
  note: 8
  note: 6
  note: 2
  note: 12
  note: 3
  note: 16
  note: 11
  note: 10
  note: 14
  note: 7
  note: 5
  note: 15
  note: 4
  note: 1
  Demux{1..12} (12 alike) : Demux  Outputs=2
  Mux15 : Mux
  Mux16 : Mux  Inputs=16
  Mux17 : Mux  Inputs=16
  Mux6 : Mux  Inputs=16
  To Workspace : ToWorkspace  VariableName=mainResults  SaveFormat=Structure With Time  SampleTime=-1
  To Workspace1 : ToWorkspace  VariableName=fullStateSTC  SaveFormat=Structure With Time  SampleTime=-1
  To Workspace2 : ToWorkspace  VariableName=HOSMO_STC  SaveFormat=Structure With Time  SampleTime=-1
  To Workspace3 : ToWorkspace  VariableName=UKF_STC  SaveFormat=Structure With Time  SampleTime=-1
  wires:
  [X2_h_HOSMO] -> Demux9/1
  [U_HOSMO] -> Demux4/1  "Total Control"
  [DL_r] -> Mux6/12  "Rear Dynamic Load"
  [z1_h] -> Mux16/7
  [z_o1] -> Mux6/1  "Front road input"
  [d2_phi] -> Mux6/8  "Pitch Acceleration"
  [z_o2] -> Mux6/2  "Rear road input"
  Demux10/1 -> Mux17/13
  Demux7/1 -> Mux17/7
  Mux17/1 -> To Workspace2/1
  [R_f] -> Mux6/13  "Front Load Ratio"
  Mux15/1 -> To Workspace1/1
  Demux7/2 -> Mux17/8
  [z2] -> Mux6/6  "Rear unsprung Displacement"
  [d_z1_h] -> Mux16/14
  [S_h_UKF] -> Demux5/1  "Sliding Surface"
  [d2_zc] -> Mux6/7  "Vertical Acceleration"
  Demux6/1 -> Mux17/5
  [S_h_HOSMO] -> Demux3/1  "Sliding Surface"
  [zc_h] -> Mux16/5
  Demux6/2 -> Mux17/6
  [U_FS_STC] -> Demux2/1  "Total Control"
  [d_zc_h] -> Mux16/10
  [d_z1] -> Mux16/13
  Demux9/1 -> Mux17/11
  [d_zc] -> Mux16/9
  [phi_h] -> Mux16/6
  Mux6/1 -> To Workspace/1
  [SL_f] -> Mux6/9  "Front Static Load"
  [X3_h_HOSMO] -> Demux11/1
  [phi] -> Mux6/4  "Pitch Motion"
  Demux11/2 -> Mux17/16
  [X1_h_HOSMO] -> Demux7/1
  [z1] -> Mux6/5  "Front unsprung Displacement"
  Demux11/1 -> Mux17/15
  [zc] -> Mux6/3  "Vertical Displacement"
  [S_FS_STC] -> Demux1/1  "Sliding Surface"
  [d_z2_h] -> Mux16/16
  Demux8/1 -> Mux17/9
  [SL_r] -> Mux6/10  "Rear Static Load"
  [z2_h] -> Mux16/8
  [d_z2] -> Mux16/15
  [X1_HOSMO] -> Demux6/1
  [d_phi] -> Mux16/11
  Demux8/2 -> Mux17/10
  [U_UKF] -> Demux12/1  "Total Control"
  [DL_f] -> Mux6/11  "Front Dynamic Load"
  Mux16/1 -> To Workspace3/1
  Demux10/2 -> Mux17/14
  [X2_HOSMO] -> Demux8/1
  Demux9/2 -> Mux17/12
  [R_r] -> Mux6/14  "Rear Load Ratio"
  [d_phi_h] -> Mux16/12
  [X3_HOSMO] -> Demux10/1
  [delta_y1] -> Mux6/15  "Front relative displacement"
  [delta_y2] -> Mux6/16  "Rear relative displacement"
  Demux1/1 -> Mux15/1
  Demux1/2 -> Mux15/2
  Demux2/1 -> Mux15/3
  Demux2/2 -> Mux15/4
  Demux3/1 -> Mux17/1
  Demux3/2 -> Mux17/2
  Demux4/1 -> Mux17/3
  Demux4/2 -> Mux17/4
  Demux12/2 -> Mux16/4
  Demux12/1 -> Mux16/3
  Demux5/2 -> Mux16/2
  Demux5/1 -> Mux16/1

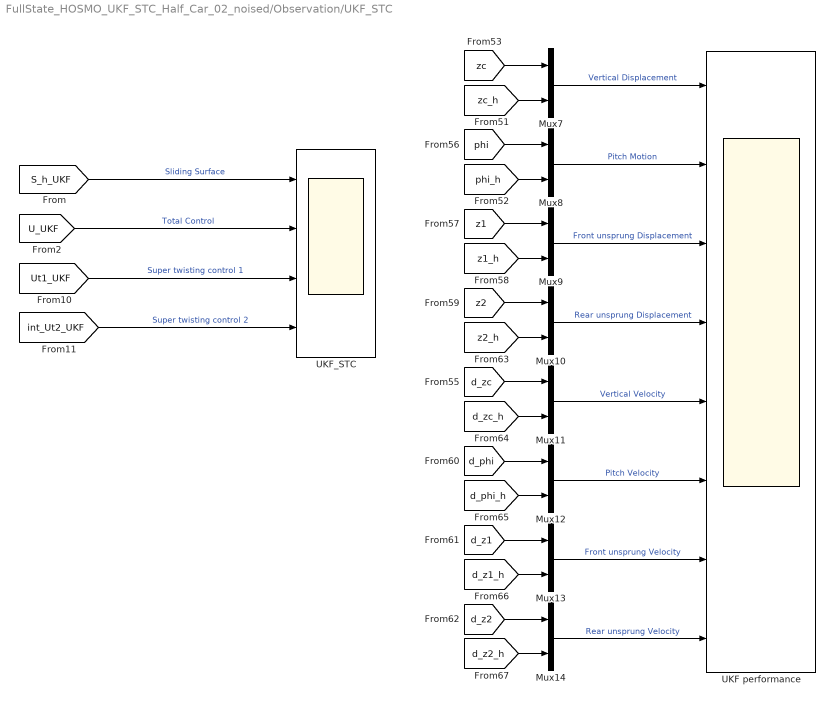
== system FullState_HOSMO_UKF_STC_Half_Car_02_noised/Observation/UKF_STC ==
  Mux{7..14} (8 alike) : Mux  Inputs=2
  UKF performance : Scope  NumInputPorts=8
  UKF_STC : Scope  NumInputPorts=4
  wires:
  Mux7/1 -> UKF performance/1  "Vertical Displacement"
  [S_h_UKF] -> UKF_STC/1  "Sliding Surface"
  [d_z1_h] -> Mux13/2
  [zc] -> Mux7/1
  Mux8/1 -> UKF performance/2  "Pitch Motion"
  [d_z1] -> Mux13/1
  [phi_h] -> Mux8/2
  [U_UKF] -> UKF_STC/2  "Total Control"
  Mux9/1 -> UKF performance/3  "Front unsprung Displacement"
  [int_Ut2_UKF] -> UKF_STC/4  "Super twisting control 2"
  [z2_h] -> Mux10/2
  [d_phi_h] -> Mux12/2
  [d_zc_h] -> Mux11/2
  Mux14/1 -> UKF performance/8  "Rear unsprung Velocity"
  [phi] -> Mux8/1
  [d_zc] -> Mux11/1
  Mux13/1 -> UKF performance/7  "Front unsprung Velocity"
  [Ut1_UKF] -> UKF_STC/3  "Super twisting control 1"
  Mux10/1 -> UKF performance/4  "Rear unsprung Displacement"
  [zc_h] -> Mux7/2
  Mux12/1 -> UKF performance/6  "Pitch Velocity"
  [d_phi] -> Mux12/1
  [z2] -> Mux10/1
  [z1_h] -> Mux9/2
  [d_z2_h] -> Mux14/2
  [d_z2] -> Mux14/1
  Mux11/1 -> UKF performance/5  "Vertical Velocity"
  [z1] -> Mux9/1

== system FullState_HOSMO_UKF_STC_Half_Car_02_noised/Unscented Kalman Filter/Simulink Function - Measurement Function ==
  SuspensionMeasurementFcn : TriggerPort  TriggerType=function-call  IsSimulinkFunction=on  FunctionName=SuspensionMeasurementFcn  VariantControl=Variant
  f(x) : MATLAB Function  TreatAsAtomicUnit=on
  x : ArgIn  DisableCoverage=on  PortDimensions=[8,1]  ArgumentName=x
  y : ArgOut  DisableCoverage=on  PortDimensions=[2,1]  ArgumentName=y
  wires:
  x/1 -> f(x)/1(X)
  f(x)/1(y) -> y/1

== system FullState_HOSMO_UKF_STC_Half_Car_02_noised/Unscented Kalman Filter/Simulink Function - State Transition Function ==
  U : Inport
  SuspensionStateFcn : TriggerPort  TriggerType=function-call  IsSimulinkFunction=on  FunctionName=SuspensionStateFcn  VariantControl=Variant
  Add : Sum
  Demux : Demux  Outputs=2
  Product : Product
  Time constant : Constant  Value=1E-4
  f(x,u) : MATLAB Function  TreatAsAtomicUnit=on
  x : ArgIn  DisableCoverage=on  PortDimensions=[8,1]  ArgumentName=x
  xNext : ArgOut  DisableCoverage=on  PortDimensions=[8,1]  ArgumentName=xNext
  wires:
  x/1 -> f(x,u)/1(X), Add/1
  Add/1 -> xNext/1
  Time constant/1 -> Product/2
  Product/1 -> Add/2
  Demux/1 -> f(x,u)/2(F1)
  Demux/2 -> f(x,u)/3(F2)
  U/1 -> Demux/1
  f(x,u)/1(Xdot) -> Product/1

== matlab function FullState_HOSMO_UKF_STC_Half_Car_02_noised/Suspension Systems/Relative Displacement & Velocity ==
  data: zc input; d_zc input; delta_y1 output; phi input; d_phi input; z1 input; d_z1 input; z2 input; delta_y2 output; d_z2 input; d_delta_y1 output; d_delta_y2 output
function [delta_y1, delta_y2, d_delta_y1, d_delta_y2] = fcn(zc, d_zc, phi, d_phi, z1, d_z1, z2, d_z2)
%% Parameters
% M = 1200; % [kg] mass of the vehicle body
% M_max = 1500; % [kg]
% M_min = 1000; % [kg]
% m_f = 100; m_r = 100; % [kg] unsprung masses of front and rear
% b_e1 = 2500; b_e2 = 2500; % [Ns/m] damping coefficient of the suspension system
% k_s1 = 15000; k_s2 = 15000; % [N/m] stiffness coefficient of the suspension system
% k_t1 = 200000; k_t2 = 200000; % [N/m] conpressibleness coefficient of the pneumatic tire
% P_s = 5*10^6; % [Pa] supply pressure
% mu = 2.32*10^8;
% C_tp = 4*10^-13; % total leakage coefficient of the piston
% V_t = 1.2*10^-3; % [m^3] total actuator volume
% V_0  = 20; % [m/s] velocity of the vehicle
% I = 600; I_max = 700; I_min = 500; % [kgm^2] mass moment of inertia
% k_nf1 = 1000; k_nr1 = 1000; % [N/m]
% b_t1 = 1000; b_t2 = 1000; % [N/m] damping coefficient of the pneumatic tire
a = 1.2; b = 1.5; % [m] distance of the suspensions to the center of mass of the vehicle body
% A = 0.006; % [m^2] ram area of the cylinder
% beta_e = 700*10^6; % [Pa] effective bulk modulus
% beta_emax = 800*10^6; % [Pa]
% beta_emin = 200*10^6; % [Pa]
%% Suspension displacements
delta_y1 = zc + a*sin(phi) - z1;
delta_y2 = zc - b*sin(phi) - z2;
d_delta_y1 = d_zc + a*d_phi*cos(phi) - d_z1;
d_delta_y2 = d_zc - b*d_phi*cos(phi) - d_z2;

== matlab function FullState_HOSMO_UKF_STC_Half_Car_02_noised/Observation/HOSMO_STC/HOSMO Errors Calculation ==
  data: zc input; d_zc input; E1 output; E2 output; E3 output; phi input; d_phi input; z1 input; d_z1 input; z2 input; d_z2 input; X1_h input; X2_h input; X3_h input; X1 output; X2 output; X3 output
function [E1, E2, E3, X1, X2, X3] = fcn(zc, d_zc, phi, d_phi, z1, d_z1, z2, d_z2, X1_h, X2_h, X3_h)
%% Parameters
M = 1200; % [kg] mass of the vehicle body
% M_max = 1500; % [kg]
% M_min = 1000; % [kg]
% m_f = 100; m_r = 100; % [kg] unsprung masses of front and rear
b_e1 = 2500; b_e2 = 2500; % [Ns/m] damping coefficient of the suspension system
k_s1 = 15000; k_s2 = 15000; % [N/m] stiffness coefficient of the suspension system
% k_t1 = 200000; k_t2 = 200000; % [N/m] conpressibleness coefficient of the pneumatic tire
% P_s = 5*10^6; % [Pa] supply pressure
% mu = 2.32*10^8;
% C_tp = 4*10^-13; % total leakage coefficient of the piston
% V_t = 1.2*10^-3; % [m^3] total actuator volume
% V_0  = 20; % [m/s] velocity of the vehicle
I = 600;
% I_max = 700; I_min = 500; % [kgm^2] mass moment of inertia
% k_nf1 = 1000; k_nr1 = 1000; % [N/m]
% b_t1 = 1000; b_t2 = 1000; % [N/m] damping coefficient of the pneumatic tire
a = 1.2; b = 1.5; % [m] distance of the suspensions to the center of mass of the vehicle body
% A = 0.006; % [m^2] ram area of the cylinder
% beta_e = 700*10^6; % [Pa] effective bulk modulus
% beta_emax = 800*10^6; % [Pa]
% beta_emin = 200*10^6; % [Pa]
%% Error Calculation
X1 = [zc; phi];
X2 = [d_zc; d_phi];
% Internal Matrices
A = [-(k_s1 + k_s2)/M, -(a*k_s1 - b*k_s2)/M; -(a*k_s1 - b*k_s2)/I, -(a^2*k_s1 + b^2*k_s2)/I];
B = [-(b_e1 + b_e2)/M, -(a*b_e1 - b*b_e2)/M; -(a*b_e1 - b*b_e2)/I, -(a^2*b_e1 + b^2*b_e2)/I];
H = A*X1 + B*X2; % actual
H_h = A*X1 + B*X2_h; % estimated
% Lumped Disturbance
d1 = (-1/M)*(-k_s1*z1 - k_s2*z2 - b_e1*d_z1 - b_e2*d_z2 + (a*k_s1 - b*k_s2)*(sin(phi)-phi) + (a*b_e1-b*b_e2)*d_phi*(cos(phi)-1));
d2 = (-1/I)*(-a*k_s1*z1 + b*k_s2*z2 - a*b_e1*d_z1 + b*b_e2*d_z2 + (a^2*k_s1 + b^2*k_s2)*(sin(phi) - phi) + (a^2*b_e1 - b^2*b_e2)*d_phi*(cos(phi)-1));
D = [d1; d2];
X3 = D + H - H_h;
% Observer estimation errors
E1 = X1 - X1_h;
E2 = X2 - X2_h;
E3 = X3 - X3_h;

== matlab function FullState_HOSMO_UKF_STC_Half_Car_02_noised/Full-state feedback STC/Full-state feedback STC ==
  data: zc input; S output; phi input; d_zc input; d_phi input; int_Ut2 input; U output; Ut1 output; Ut2 output; C1 input; Lambda1 input; Lambda2 input
function [S, U, Ut1, Ut2] = fcn(zc, phi, d_zc, d_phi, int_Ut2, C1, Lambda1, Lambda2)
%% Parameters
M = 1200; % [kg] mass of the vehicle body
% M_max = 1500; % [kg]
% M_min = 1000; % [kg]
b_e1 = 2500; b_e2 = 2500; % [Ns/m] damping coefficient of the suspension system
k_s1 = 15000; k_s2 = 15000; % [N/m] stiffness coefficient of the suspension system
I = 600; % [kgm^2] mass moment of inertia
% I_max = 700; I_min = 500;
a = 1.2; b = 1.5; % [m] distance of the suspensions to the center of mass of the vehicle body
%% Control-oriented System Dynamics
% d_X1 = X2;
% d_X2 = H + G*U + D
X1 = [zc; phi];
X2 = [d_zc; d_phi];
% Internal Matrices
A = [-(k_s1 + k_s2)/M, -(a*k_s1 - b*k_s2)/M; -(a*k_s1 - b*k_s2)/I, -(a^2*k_s1 + b^2*k_s2)/I];
B = [-(b_e1 + b_e2)/M, -(a*b_e1 - b*b_e2)/M; -(a*b_e1 - b*b_e2)/I, -(a^2*b_e1 + b^2*b_e2)/I];
H = A*X1 + B*X2; % actual
% Control Matrix
G = [1/M, 1/M; a/I, -b/I];
% Sliding surface
S = C1*X1 + X2;
% Control law
Ut1 = Lambda1.*nthroot(abs(S),2).*sign(S);
Ut2 = Lambda2.*sign(S);
U = G\(-C1.*X2 - H - Ut1 - int_Ut2);

== matlab function FullState_HOSMO_UKF_STC_Half_Car_02_noised/Unscented Kalman Filter/Simulink Function - Measurement Function/f(x) ==
  data: X input; y output
function y = fy(X)
%% Parameters
% M = 1200; % [kg] mass of the vehicle body
% M_max = 1500; % [kg]
% M_min = 1000; % [kg]
% m_f = 100; m_r = 100; % [kg] unsprung masses of front and rear
% b_e1 = 2500; b_e2 = 2500; % [Ns/m] damping coefficient of the suspension system
% k_s1 = 15000; k_s2 = 15000; % [N/m] stiffness coefficient of the suspension system
% k_t1 = 200000; k_t2 = 200000; % [N/m] conpressibleness coefficient of the pneumatic tire
% P_s = 5*10^6; % [Pa] supply pressure
% mu = 2.32*10^8;
% C_tp = 4*10^-13; % total leakage coefficient of the piston
% V_t = 1.2*10^-3; % [m^3] total actuator volume
% V_0  = 20; % [m/s] velocity of the vehicle
% I = 600; I_max = 700; I_min = 500; % [kgm^2] mass moment of inertia
% k_nf1 = 1000; k_nr1 = 1000; % [N/m]
% b_t1 = 1000; b_t2 = 1000; % [N/m] damping coefficient of the pneumatic tire
a = 1.2; b = 1.5; % [m] distance of the suspensions to the center of mass of the vehicle body
% A = 0.006; % [m^2] ram area of the cylinder
% beta_e = 700*10^6; % [Pa] effective bulk modulus
% beta_emax = 800*10^6; % [Pa]
% beta_emin = 200*10^6; % [Pa]
%% Suspension displacements
%
% X = [zc, d_zc, phi, d_phi, z1, d_z1, z2, d_z2]'
% Xdot = [d_zc, d2_zc, d_phi, d2_phi, d_z1, d2_z1, d_z2, d2_z2]'
%
delta_y1 = X(1) + a*sin(X(3)) - X(5);
delta_y2 = X(1) - b*sin(X(3)) - X(7);
%
y = [delta_y1; delta_y2];

== matlab function FullState_HOSMO_UKF_STC_Half_Car_02_noised/Unscented Kalman Filter/Simulink Function - State Transition Function/f(x,u) ==
  data: X input; F1 input; F2 input; Xdot output
function Xdot = fx(X,F1,F2)
%% Parameters
M = 1200; % [kg] mass of the vehicle body
% M_max = 1500; % [kg]
% M_min = 1000; % [kg]
m_f = 100; m_r = 100; % [kg] unsprung masses of front and rear
b_e1 = 2500; b_e2 = 2500; % [Ns/m] damping coefficient of the suspension system
k_s1 = 15000; k_s2 = 15000; % [N/m] stiffness coefficient of the suspension system
I = 600; % [kgm^2] mass moment of inertia
% I_max = 700; I_min = 500;
a = 1.2; b = 1.5; % [m] distance of the suspensions to the center of mass of the vehicle body
%% Suspension displacements
%
% X = [zc, d_zc, phi, d_phi, z1, d_z1, z2, d_z2]'
% Xdot = [d_zc, d2_zc, d_phi, d2_phi, d_z1, d2_z1, d_z2, d2_z2]'
%
delta_y1 = X(1) + a*sin(X(3)) - X(5);
delta_y2 = X(1) - b*sin(X(3)) - X(7);
d_delta_y1 = X(2) + a*X(4)*cos(X(3)) - X(6);
d_delta_y2 = X(2) - b*X(4)*cos(X(3)) - X(8);
%% Differential Equations - Unsprung mass displacements
%
d2_z1 = (1/m_f)*(k_s1*delta_y1 + b_e1*d_delta_y1 - F1);
%
d2_z2 = (1/m_r)*(k_s2*delta_y2 + b_e2*d_delta_y2 - F2);
%% Active Suspension subsystems
phi_1 = k_s1*delta_y1 + k_s2*delta_y2 + b_e1*d_delta_y1 + b_e2*d_delta_y2;
phi_2 = a*(k_s1*delta_y1 + b_e1*d_delta_y1) - b*(k_s2*delta_y2 + b_e2*d_delta_y2);
%
d2_zc = (1/M)*(-phi_1 + F1 + F2);
%
d2_phi = (1/I)*(-phi_2 + a*F1 - b*F2);
%
Xdot = zeros(size(X));
%
Xdot(1) = X(2);
Xdot(2) = d2_zc;
Xdot(3) = X(4);
Xdot(4) = d2_phi;
Xdot(5) = X(6);
Xdot(6) = d2_z1;
Xdot(7) = X(8);
Xdot(8) = d2_z2;

== matlab function FullState_HOSMO_UKF_STC_Half_Car_02_noised/Observation/OVERALL/Load Calculation ==
  data: z1 input; SL_f output; z2 input; d_z1 input; d_z2 input; z_o1 input; z_o2 input; d_z_o1 input; d_z_o2 input; SL_r output; DL_f output; DL_r output; R_f output; R_r output
function [SL_f, SL_r, DL_f, DL_r, R_f, R_r] = fcn(z1, z2, d_z1, d_z2, z_o1, z_o2, d_z_o1, d_z_o2)
%% Parameters
M = 1200; % [kg] mass of the vehicle body
% M_max = 1500; % [kg]
% M_min = 1000; % [kg]
m_f = 100; m_r = 100; % [kg] unsprung masses of front and rear
% b_e1 = 2500; b_e2 = 2500; % [Ns/m] damping coefficient of the suspension system
% k_s1 = 15000; k_s2 = 15000; % [N/m] stiffness coefficient of the suspension system
k_t1 = 200000; k_t2 = 200000; % [N/m] conpressibleness coefficient of the pneumatic tire
% P_s = 5*10^6; % [Pa] supply pressure
% mu = 2.32*10^8;
% C_tp = 4*10^-13; % total leakage coefficient of the piston
% V_t = 1.2*10^-3; % [m^3] total actuator volume
% V_0  = 20; % [m/s] velocity of the vehicle
% I = 600; % [kgm^2] mass moment of inertia
% I_max = 700; I_min = 500;
% k_nf1 = 1000; k_nr1 = 1000; % [N/m]
b_t1 = 1000; b_t2 = 1000; % [N/m] damping coefficient of the pneumatic tire
a = 1.2; b = 1.5; % [m] distance of the suspensions to the center of mass of the vehicle body
% A = 0.006; % [m^2] ram area of the cylinder
% beta_e = 700*10^6; % [Pa] effective bulk modulus
% beta_emax = 800*10^6; % [Pa]
% beta_emin = 200*10^6; % [Pa]
g = 9.81; % [m/s^2] gravitational acceleration
% Dynamic Loads
DL_f = k_t1*(z1 - z_o1) + b_t1*(d_z1 - d_z_o1);
DL_r = k_t2*(z2 - z_o2) + b_t2*(d_z2 - d_z_o2);
% Static Loads
SL_f = (M*g*b + m_f*g*(a+b))/(a+b);
SL_r = (M + m_f + m_r)*g - SL_f;
% Ratios
R_f = abs(DL_f/SL_f);
R_r = abs(DL_r/SL_r);

== matlab function FullState_HOSMO_UKF_STC_Half_Car_02_noised/UKF based STC/STC ==
  data: zc_h input; d_zc_h input; phi_h input; d_phi_h input; z1_h input; S_h output; z2_h input; d_z1_h input; d_z2_h input; int_Ut2 input; C1 input; Lambda1 input; Lambda2 input; U output; Ut1 output; Ut2 output
function [S_h, U, Ut1, Ut2] = fcn(zc_h, d_zc_h, phi_h, d_phi_h, z1_h, z2_h, d_z1_h, d_z2_h, int_Ut2, C1, Lambda1, Lambda2)
%% Parameters
M = 1200; % [kg] mass of the vehicle body
% M_max = 1500; % [kg]
% M_min = 1000; % [kg]
b_e1 = 2500; b_e2 = 2500; % [Ns/m] damping coefficient of the suspension system
k_s1 = 15000; k_s2 = 15000; % [N/m] stiffness coefficient of the suspension system
I = 600;
% I_max = 700; I_min = 500; % [kgm^2] mass moment of inertia
a = 1.2; b = 1.5; % [m] distance of the suspensions to the center of mass of the vehicle body
%% State-space model
X1_h = [zc_h; phi_h];
X2_h = [d_zc_h; d_phi_h];
% Dynamic matrices
delta_y1_h = zc_h + a*sin(phi_h) - z1_h;
delta_y2_h = zc_h - b*sin(phi_h) - z2_h;
d_delta_y1_h = d_zc_h + a*d_phi_h*cos(phi_h) - d_z1_h;
d_delta_y2_h = d_zc_h - b*d_phi_h*cos(phi_h) - d_z2_h;
%
Phi1_h = k_s1*delta_y1_h + k_s2*delta_y2_h + b_e1*d_delta_y1_h + b_e2*d_delta_y2_h;
Phi2_h = a*(k_s1*delta_y1_h + b_e1*d_delta_y1_h) - b*(k_s2*delta_y2_h + b_e2*d_delta_y2_h);
%
H_h = [(-1/M)*Phi1_h; (-1/I)*Phi2_h];
G = [1/M, 1/M; a/I, -b/I];
% State-space form
% d_X1_h = X2_h;
% d_X2_h = H_h + G*U;
% Sliding Surface
S_h = C1.*X1_h + X2_h;
% Super twisting control components
Ut1 = Lambda1.*nthroot(abs(S_h),2).*sign(S_h);
% Ut1 = Lambda1.*sqrt(abs(S_h)).*sign(S_h);
Ut2 = Lambda2.*sign(S_h);
% Control law
U = (G^-1)*(-C1.*X2_h - H_h - Ut1 - int_Ut2);

== matlab function FullState_HOSMO_UKF_STC_Half_Car_02_noised/HOSMO/HOSMO_2States ==
  data: zc input; d_X1_h output; d_X2_h output; d_X3_h output; phi input; X1_h input; X2_h input; X3_h input; U input; K1 input; K2 input; K3 input
function [d_X1_h, d_X2_h, d_X3_h] = fcn(zc, phi, X1_h, X2_h, X3_h, U, K1, K2, K3)
%% Parameters
M = 1200; % [kg] mass of the vehicle body
% M_max = 1500; % [kg]
% M_min = 1000; % [kg]
b_e1 = 2500; b_e2 = 2500; % [Ns/m] damping coefficient of the suspension system
k_s1 = 15000; k_s2 = 15000; % [N/m] stiffness coefficient of the suspension system
I = 600; % [kgm^2] mass moment of inertia
% I_max = 700; I_min = 500;
a = 1.2; b = 1.5; % [m] distance of the suspensions to the center of mass of the vehicle body
%% Control-oriented System Dynamics
% d_X1 = X2;
% d_X2 = H + G*U + D
X1 = [zc; phi];
% Internal Matrices
A = [-(k_s1 + k_s2)/M, -(a*k_s1 - b*k_s2)/M; -(a*k_s1 - b*k_s2)/I, -(a^2*k_s1 + b^2*k_s2)/I];
B = [-(b_e1 + b_e2)/M, -(a*b_e1 - b*b_e2)/M; -(a*b_e1 - b*b_e2)/I, -(a^2*b_e1 + b^2*b_e2)/I];
% H = A*X1 + B*X2; % actual
H_h = A*X1 + B*X2_h; % estimated
% Control Matrix
G = [1/M, 1/M; a/I, -b/I];
% Lumped Disturbance
% d1 = (-1/M)*(-k_s1*z1 - k_s2*z2 - b_e1*d_z1 - b_e2*d_z2 + (a*k_s1 - b*k_s2)*(sin(phi)-phi) + (a*b_e1-b*b_e2)*d_phi*(cos(phi)-1));
% d2 = (-1/I)*(-a*k_s1*z1 + b*k_s2*z2 - a*b_e1*d_z1 + b*b_e2*d_z2 + (a^2*k_s1 + b^2*k_s2)*(sin(phi) - phi) + (a^2*b_e1 - b^2*b_e2)*d_phi*(cos(phi)-1));
% D = [d1; d2];
% Observer estimation errors
E1 = X1 - X1_h;
% E2 = X2 - X2_h;
% E3 = D - X3_h + H - H_h;
% Correction terms
Z1 = K1.*nthroot(abs(E1).^2,3).*sign(E1);
Z2 = K2.*nthroot(abs(E1).^1,3).*sign(E1);
Z3 = K3.*sign(E1);
% Observer
d_X1_h = X2_h + Z1;
d_X2_h = X3_h + H_h + G*U + Z2;
d_X3_h = Z3;

== matlab function FullState_HOSMO_UKF_STC_Half_Car_02_noised/Suspension Systems/Dynamics ==
  data: d2_zc output; d2_phi output; zc input; d2_z1 output; d_zc input; phi input; d_phi input; z1 input; z2 input; d_z1 input; d_z2 input; z_o1 input; z_o2 input; dz_o1 input; dz_o2 input; F1 input; F2 input; d2_z2 output
function [d2_zc, d2_phi, d2_z1, d2_z2] = fcn(zc, d_zc, phi, d_phi, z1, z2, d_z1, d_z2, z_o1, z_o2, dz_o1, dz_o2, F1, F2)
%% Parameters
M = 1200; % [kg] mass of the vehicle body
% M_max = 1500; % [kg]
% M_min = 1000; % [kg]
m_f = 100; m_r = 100; % [kg] unsprung masses of front and rear
b_e1 = 2500; b_e2 = 2500; % [Ns/m] damping coefficient of the suspension system
k_s1 = 15000; k_s2 = 15000; % [N/m] stiffness coefficient of the suspension system
k_t1 = 200000; k_t2 = 200000; % [N/m] conpressibleness coefficient of the pneumatic tire
% P_s = 5*10^6; % [Pa] supply pressure
% mu = 2.32*10^8;
% C_tp = 4*10^-13; % total leakage coefficient of the piston
% V_t = 1.2*10^-3; % [m^3] total actuator volume
% V_0  = 20; % [m/s] velocity of the vehicle
I = 600; % [kgm^2] mass moment of inertia
% I_max = 700; I_min = 500;
% k_nf1 = 1000; k_nr1 = 1000; % [N/m]
b_t1 = 1000; b_t2 = 1000; % [N/m] damping coefficient of the pneumatic tire
a = 1.2; b = 1.5; % [m] distance of the suspensions to the center of mass of the vehicle body
% A = 0.006; % [m^2] ram area of the cylinder
% beta_e = 700*10^6; % [Pa] effective bulk modulus
% beta_emax = 800*10^6; % [Pa]
% beta_emin = 200*10^6; % [Pa]
%% Suspension displacements
delta_y1 = zc + a*sin(phi) - z1;
delta_y2 = zc - b*sin(phi) - z2;
d_delta_y1 = d_zc + a*d_phi*cos(phi) - d_z1;
d_delta_y2 = d_zc - b*d_phi*cos(phi) - d_z2;
%% Differential Equations - Unsprung mass displacements
d2_z1 = (1/m_f)*(k_s1*delta_y1 + b_e1*d_delta_y1 - k_t1*(z1 - z_o1) - b_t1*(d_z1 - dz_o1) - F1);
d2_z2 = (1/m_r)*(k_s2*delta_y2 + b_e2*d_delta_y2 - k_t2*(z2 - z_o2) - b_t2*(d_z2 - dz_o2) - F2);
%% Active Suspension subsystems
phi_1 = k_s1*delta_y1 + k_s2*delta_y2 + b_e1*d_delta_y1 + b_e2*d_delta_y2;
phi_2 = a*(k_s1*delta_y1 + b_e1*d_delta_y1) - b*(k_s2*delta_y2 + b_e2*d_delta_y2);
%
d2_zc = (1/M)*(-phi_1 + F1 + F2);
d2_phi = (1/I)*(-phi_2 + a*F1 - b*F2);

== matlab function FullState_HOSMO_UKF_STC_Half_Car_02_noised/Road Profile/Road profile ==
  data: t input; z_o1 output; dz_o1 output; z_o2 output; dz_o2 output
function [z_o1, dz_o1, z_o2, dz_o2] = fcn(t)
%
V_0  = 20; % [m/s] velocity of the vehicle
a = 1.2; b = 1.5; % [m] distance of the suspensions to the center of mass of the vehicle body
%
h_b = 0.02;
dt = (a+b)/V_0;
if t >= 1 && t <= 1.25
    z_o1 = h_b*(1-cos(6*pi*t))/2;
    dz_o1 = h_b*(1+6*pi*sin(6*pi*t))/2;
else
    z_o1 = 0;
    dz_o1 = 0;
end
%
if t >= 1+dt && t <= 1.25+dt
    z_o2 = h_b*(1-cos(6*pi*t))/2;
    dz_o2 = h_b*(1+6*pi*sin(6*pi*t))/2;
else
    z_o2 = 0;
    dz_o2 = 0;
end

== matlab function FullState_HOSMO_UKF_STC_Half_Car_02_noised/HOSMO based STC/HOSMO based STC ==
  data: zc input; S_h output; phi input; X1_h input; X2_h input; X3_h input; int_Ut2 input; C1 input; K2 input; Lambda1 input; Lambda2 input; U output; Ut1 output; Ut2 output
function [S_h, U, Ut1, Ut2] = fcn(zc, phi, X1_h, X2_h, X3_h, int_Ut2, C1, K2, Lambda1, Lambda2)
%% Parameters
M = 1200; % [kg] mass of the vehicle body
% M_max = 1500; % [kg]
% M_min = 1000; % [kg]
b_e1 = 2500; b_e2 = 2500; % [Ns/m] damping coefficient of the suspension system
k_s1 = 15000; k_s2 = 15000; % [N/m] stiffness coefficient of the suspension system
I = 600; % [kgm^2] mass moment of inertia
% I_max = 700; I_min = 500;
a = 1.2; b = 1.5; % [m] distance of the suspensions to the center of mass of the vehicle body
%% Control-oriented System Dynamics
% d_X1 = X2;
% d_X2 = H + G*U + D
X1 = [zc; phi];
% Internal Matrices
A = [-(k_s1 + k_s2)/M, -(a*k_s1 - b*k_s2)/M; -(a*k_s1 - b*k_s2)/I, -(a^2*k_s1 + b^2*k_s2)/I];
B = [-(b_e1 + b_e2)/M, -(a*b_e1 - b*b_e2)/M; -(a*b_e1 - b*b_e2)/I, -(a^2*b_e1 + b^2*b_e2)/I];
% H = A*X1 + B*X2; % actual
H_h = A*X1 + B*X2_h; % estimated
% Control Matrix
G = [1/M, 1/M; a/I, -b/I];
% Lumped Disturbance
% d1 = (-1/M)*(-k_s1*z1 - k_s2*z2 - b_e1*d_z1 - b_e2*d_z2 + (a*k_s1 - b*k_s2)*(sin(phi)-phi) + (a*b_e1-b*b_e2)*d_phi*(cos(phi)-1));
% d2 = (-1/I)*(-a*k_s1*z1 + b*k_s2*z2 - a*b_e1*d_z1 + b*b_e2*d_z2 + (a^2*k_s1 + b^2*k_s2)*(sin(phi) - phi) + (a^2*b_e1 - b^2*b_e2)*d_phi*(cos(phi)-1));
% D = [d1; d2];
% Observer estimation errors
E1 = X1 - X1_h;
% E2 = X2 - X2_h;
% E3 = D - X3_h + H - H_h;
% Correction terms
% Z1 = K1.*nthroot(abs(E1).^2,3).*sign(E1);
Z2 = K2.*nthroot(abs(E1),3).*sign(E1);
%
% Z2 = [K2*nthroot(abs(E1(1)),3)*sign(E1(1)); K2*nthroot(abs(E1(2)),3)*sign(E1(2))];
% Z3 = K3.*sign(E1);
% Sliding surface
S_h = C1.*X1 + X2_h;
% S_h = diag([C1,C1])*X1 + X2_h;
% Control law
Ut1 = Lambda1.*nthroot(abs(S_h),2).*sign(S_h);
Ut2 = Lambda2.*sign(S_h);
U = G\(-C1.*X2_h - H_h - Z2 - X3_h - Ut1 - int_Ut2);
% U = G\(-diag([C1,C1])*X2_h - H_h - Z2 - X3_h - Ut1 - int_Ut2);
